simulink model "hwTarget"  (R2020b)
settings: Solver=VariableStepAuto  StartTime=0.0  StopTime=Ts  RelTol=1e-3
InitFcn:
  | evalin('base','pixelcontrolbus');
  | 
  | ROWS = 480;
  | COLS = 752;
  | 
  | OFFSET = 3;
  | imagesToRead = 20;
  | Ts = (imagesToRead + OFFSET) * 2;
  | 
  | inputNums = [1:imagesToRead];
  | 
  | MagThrL = 7;
  | MagThrS = 3;
  | SegMaxLength = 630;
  | 
  | NUM_OF_BITS = 32;
  | MSB = NUM_OF_BITS-1;
  | cap_1 = fixdt(0,NUM_OF_BITS,NUM_OF_BITS-1);
  | cap_2 = fixdt(0,NUM_OF_BITS,NUM_OF_BITS-2);
  | 
  | CORDIC_LUT_DT_1 = fixdt(1, NUM_OF_BITS, NUM_OF_BITS-2);
  | CORDIC_LUT_DT_2 = fixdt(1, NUM_OF_BITS, NUM_OF_BITS-1);
  | CORDIC_LUT_DT_3 = fixdt(1, NUM_OF_BITS, NUM_OF_BITS);
  | CORDIC_LUT_DT_4 = fixdt(1, NUM_OF_BITS, NUM_OF_BITS+1);
  | CORDIC_LUT_DT_5 = fixdt(1, NUM_OF_BITS, NUM_OF_BITS+1);
  | CORDIC_LUT_DT_6 = fixdt(1, NUM_OF_BITS, NUM_OF_BITS+2);
  | CORDIC_LUT_DT_7 = fixdt(1, NUM_OF_BITS, NUM_OF_BITS+3);
  | CORDIC_LUT_DT_8 = fixdt(1, NUM_OF_BITS, NUM_OF_BITS+4);
  | CORDIC_LUT_DT_9 = fixdt(1, NUM_OF_BITS, NUM_OF_BITS+5);
  | CORDIC_LUT_DT_10 = fixdt(1, NUM_OF_BITS, NUM_OF_BITS+6);
  | CORDIC_LUT_DT_11 = fixdt(1, NUM_OF_BITS, NUM_OF_BITS+7);
  | CORDIC_LUT_DT_12 = fixdt(1, NUM_OF_BITS, NUM_OF_BITS+8);
  | 
  | RGB_DT = fixdt(0, 24, 0);
  | GRAY_DT = fixdt(0, 8, 0);
  | THETA_DT = fixdt(1, 16, 13);
  | MAG_DT = fixdt(0, 16, 15);
  | KIRCH_DT = fixdt(0, 12, 0);
undefined symbols (not defined in the file or in its folder): bufferInit, bufferSize
libraries: hdlsllib x86, simulink x6, visionhdlstatistics x4, visionhdlio x2, visionhdlutilities x1
(part 1 of 3)
settings Model: Creator=tyson  LastModifiedBy=tyson

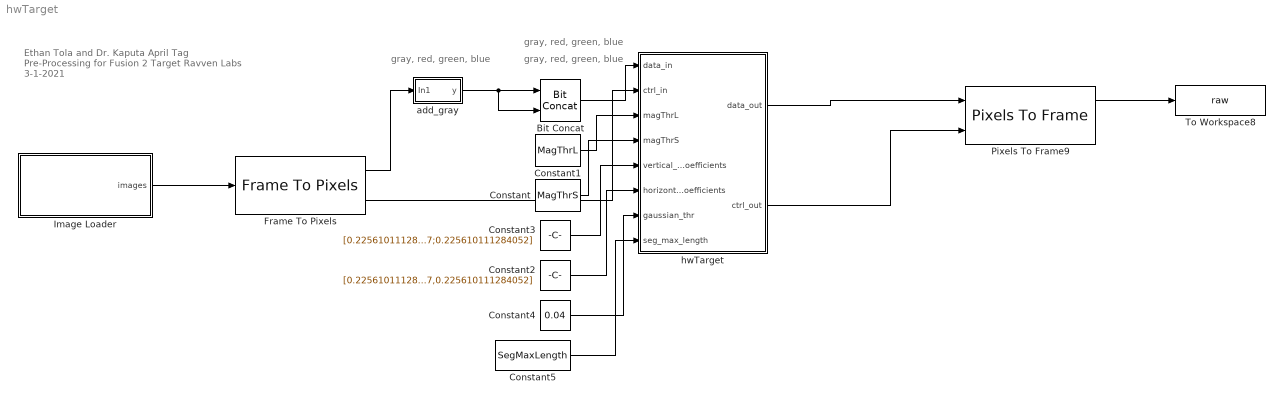
== system hwTarget ==
  note: Ethan Tola and Dr. Kaputa
      | April Tag Pre-Processing for Fusion 2 Target
      | Ravven Labs
      | 3-1-2021
  note: gray, red, green, blue
  note: gray, red, green, blue
  note: gray, red, green, blue
  Bit Concat : hdlsllib/Logic and Bit Operations/Bit Concat  numInputs=2
  Constant : Constant  Value=MagThrS  OutDataTypeStr=Inherit: Inherit via back propagation  SampleTime=-1
  Constant1 : Constant  Value=MagThrL  OutDataTypeStr=Inherit: Inherit via back propagation  SampleTime=-1
  Constant2 : Constant  Value=[0.225610111284052,0.548779777431897,0.225610111284052]  OutDataTypeStr=Inherit: Inherit via back propagation  SampleTime=-1
  Constant3 : Constant  Value=[0.225610111284051;0.548779777431897;0.225610111284052]  OutDataTypeStr=Inherit: Inherit via back propagation  SampleTime=-1
  Constant4 : Constant  Value=0.04  OutDataTypeStr=Inherit: Inherit via back propagation  SampleTime=-1
  Constant5 : Constant  Value=SegMaxLength
  Frame To Pixels : visionhdlio/Frame To Pixels  NumComponents=3  NumPixels=1  VideoFormat=Custom  ActivePixelsPerLine=752  ActiveVideoLines=480  TotalPixelsPerLine=752  TotalVideoLines=480  StartingActiveLine=1  FrontPorch=0  SampleTime=0
      settings: SourceProductName=Vision HDL Toolbox
  Image Loader : Subsystem
  Pixels To Frame9 : visionhdlio/Pixels To Frame  NumComponents=1  NumPixels=1  VideoFormat=Custom  ActivePixelsPerLine=752  ActiveVideoLines=480  TotalPixelsPerLine=752  TotalVideoLines=480
      settings: SourceProductBaseCode=VT
  To Workspace8 : ToWorkspace  VariableName=raw  SaveFormat=Timeseries  SampleTime=-1
  add_gray : Subsystem
  hwTarget : Subsystem  TreatAsAtomicUnit=on
  wires:
  Frame To Pixels/1 -> add_gray/1(In1)
  Bit Concat/1 -> hwTarget/1(data_in)
  hwTarget/1(data_out) -> Pixels To Frame9/1
  add_gray/1(y) -> Bit Concat/2, Bit Concat/1
  hwTarget/2(ctrl_out) -> Pixels To Frame9/2
  Frame To Pixels/2 -> hwTarget/2(ctrl_in)
  Pixels To Frame9/1 -> To Workspace8/1
  Image Loader/1(images) -> Frame To Pixels/1
  Constant1/1 -> hwTarget/3(magThrL)
  Constant/1 -> hwTarget/4(magThrS)
  Constant3/1 -> hwTarget/5(vertical_coefficients)
  Constant2/1 -> hwTarget/6(horizontal_coefficients)
  Constant4/1 -> hwTarget/7(gaussian_thr)
  Constant5/1 -> hwTarget/8(seg_max_length)

== system hwTarget/Image Loader ==
  Clock : Clock
  MATLAB Function : MATLAB Function  TreatAsAtomicUnit=on  SystemSampleTime=1
  images : Outport
  wires:
  Clock/1 -> MATLAB Function/1(simTime)
  MATLAB Function/1(images) -> images/1

== system hwTarget/add_gray ==
  note: Grayscale = (R * 0.25) + (G * 0.5) + (B * 0.125)
  In1 : Inport
  Bit Concat : hdlsllib/Logic and Bit Operations/Bit Concat  numInputs=4
  Demux : Demux  Outputs=3
  Shift Arithmetic3 : ArithShift  BitShiftNumber=1  BitShiftDirection=Right
  Shift Arithmetic4 : ArithShift  BitShiftNumber=2  BitShiftDirection=Right
  Shift Arithmetic5 : ArithShift  BitShiftNumber=3  BitShiftDirection=Right
  Sum : Sum  Inputs=+++  OutDataTypeStr=uint8
  y : Outport
  wires:
  Bit Concat/1 -> y/1
  In1/1 -> Demux/1
  Demux/2 -> Shift Arithmetic3/1, Bit Concat/3
  Demux/1 -> Shift Arithmetic4/1, Bit Concat/2
  Demux/3 -> Shift Arithmetic5/1, Bit Concat/4
  Sum/1 -> Bit Concat/1
  Shift Arithmetic4/1 -> Sum/1
  Shift Arithmetic3/1 -> Sum/2
  Shift Arithmetic5/1 -> Sum/3

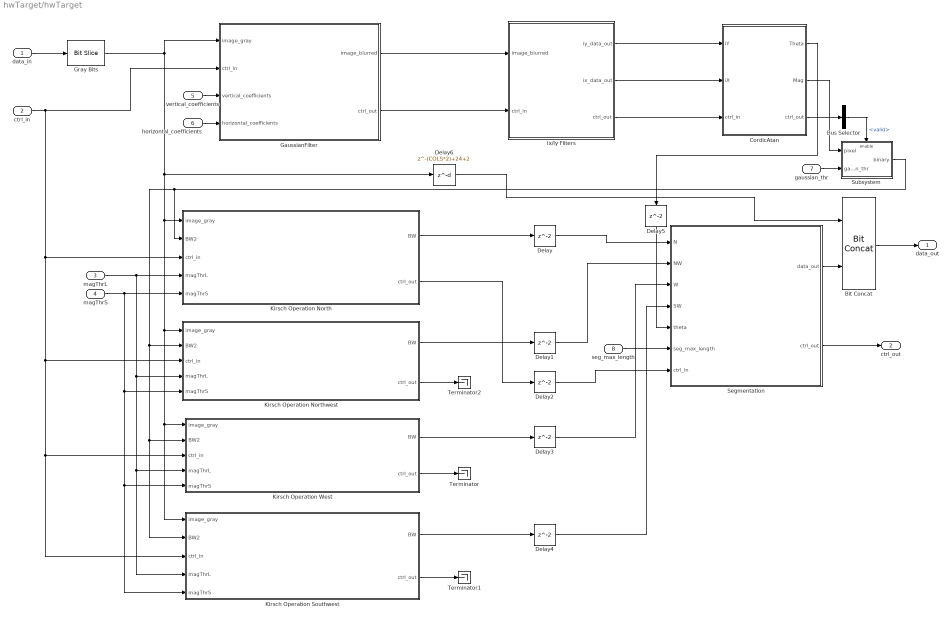
== system hwTarget/hwTarget ==
  data_in : Inport
  ctrl_in : Inport  Port=2
  magThrL : Inport  Port=3
  magThrS : Inport  Port=4
  vertical_coefficients : Inport  Port=5
  horizontal_coefficients : Inport  Port=6
  gaussian_thr : Inport  Port=7
  seg_max_length : Inport  Port=8
  Bit Concat : hdlsllib/Logic and Bit Operations/Bit Concat  numInputs=2
  Bus Selector : BusSelector  OutputSignals=valid
  CordicAtan : Subsystem
  Delay{,1..5} (6 alike) : Delay
  Delay6 : Delay  DelayLength=(COLS*2)+24+2
  GaussianFilter : Subsystem
  Gray Bits : hdlsllib/Logic and Bit Operations/Bit Slice  lidx=31  ridx=24
      settings: SourceProductBaseCode=SL
  Ix/Iy Filters : Subsystem
  Kirsch Operation North : Subsystem
  Kirsch Operation Northwest : Subsystem
  Kirsch Operation Southwest : Subsystem
  Kirsch Operation West : Subsystem
  Segmentation : Subsystem
  Subsystem : Subsystem
  Terminator : Terminator
  Terminator1 : Terminator
  Terminator2 : Terminator
  data_out : Outport
  ctrl_out : Outport  Port=2
  wires:
  Ix/Iy Filters/3(ctrl_out) -> CordicAtan/3(ctrl_in)
  GaussianFilter/2(ctrl_out) -> Ix/Iy Filters/2(ctrl_in)
  GaussianFilter/1(image_blurred) -> Ix/Iy Filters/1(image_blurred)
  Ix/Iy Filters/2(ix_data_out) -> CordicAtan/2(iX)
  Ix/Iy Filters/1(iy_data_out) -> CordicAtan/1(iY)
  data_in/1 -> Gray Bits/1
  CordicAtan/2(Mag) -> Subsystem/1(pixel)
  Bus Selector/1 -> Subsystem/Enable  "<valid>"
  ctrl_in/1 -> Kirsch Operation Southwest/3(ctrl_in), Kirsch Operation West/3(ctrl_in), Kirsch Operation Northwest/3(ctrl_in), Kirsch Operation North/3(ctrl_in), GaussianFilter/2(ctrl_in)
  Gray Bits/1 -> Delay6/1, Kirsch Operation Southwest/1(image_gray), Kirsch Operation West/1(image_gray), Kirsch Operation Northwest/1(image_gray), Kirsch Operation North/1(image_gray), GaussianFilter/1(image_gray)
  Subsystem/1(binary) -> Kirsch Operation North/2(BW2), Kirsch Operation Southwest/2(BW2), Kirsch Operation West/2(BW2), Kirsch Operation Northwest/2(BW2)
  CordicAtan/1(Theta) -> Delay5/1
  CordicAtan/3(ctrl_out) -> Bus Selector/1
  magThrL/1 -> Kirsch Operation Southwest/4(magThrL), Kirsch Operation West/4(magThrL), Kirsch Operation Northwest/4(magThrL), Kirsch Operation North/4(magThrL)
  magThrS/1 -> Kirsch Operation Southwest/5(magThrS), Kirsch Operation West/5(magThrS), Kirsch Operation Northwest/5(magThrS), Kirsch Operation North/5(magThrS)
  vertical_coefficients/1 -> GaussianFilter/3(vertical_coefficients)
  horizontal_coefficients/1 -> GaussianFilter/4(horizontal_coefficients)
  gaussian_thr/1 -> Subsystem/2(gaussian_thr)
  Kirsch Operation North/1(BW) -> Delay/1
  Kirsch Operation Northwest/1(BW) -> Delay1/1
  Kirsch Operation West/1(BW) -> Delay3/1
  Kirsch Operation Southwest/1(BW) -> Delay4/1
  Kirsch Operation North/2(ctrl_out) -> Delay2/1
  Delay/1 -> Segmentation/1(N)
  Delay1/1 -> Segmentation/2(NW)
  Delay2/1 -> Segmentation/7(ctrl_in)
  Delay3/1 -> Segmentation/3(W)
  Delay4/1 -> Segmentation/4(SW)
  Delay5/1 -> Segmentation/5(theta)
  Segmentation/2(ctrl_out) -> ctrl_out/1
  Kirsch Operation West/2(ctrl_out) -> Terminator/1
  Kirsch Operation Southwest/2(ctrl_out) -> Terminator1/1
  Kirsch Operation Northwest/2(ctrl_out) -> Terminator2/1
  Bit Concat/1 -> data_out/1
  Segmentation/1(data_out) -> Bit Concat/2
  Delay6/1 -> Bit Concat/1
  seg_max_length/1 -> Segmentation/6(seg_max_length)

== system hwTarget/hwTarget/CordicAtan ==
  iY : Inport
  iX : Inport  Port=2
  ctrl_in : Inport  Port=3
  Bus Selector : BusSelector  OutputSignals=valid
  CORDIC Algorithm : Subsystem
  Delay32 : Delay  DelayLength=14
  Theta : Outport
  Mag : Outport  Port=2
  ctrl_out : Outport  Port=3
  wires:
  Delay32/1 -> ctrl_out/1
  iY/1 -> CORDIC Algorithm/1(In1)
  iX/1 -> CORDIC Algorithm/2(In2)
  CORDIC Algorithm/1(Out1) -> Theta/1
  CORDIC Algorithm/2(Out2) -> Mag/1
  ctrl_in/1 -> Delay32/1, Bus Selector/1
  Bus Selector/1 -> CORDIC Algorithm/Enable  "<valid>"

== system hwTarget/hwTarget/GaussianFilter ==
  image_gray : Inport
  ctrl_in : Inport  Port=2
  vertical_coefficients : Inport  Port=3
  horizontal_coefficients : Inport  Port=4
  Bus Selector : BusSelector  OutputSignals=valid
  Data Type Duplicate : DataTypeDuplicate  NumInputPorts=3
  Delay1 : Delay  DelayLength=4
  Delay2 : Delay  DelayLength=4
  Normalize : Gain  Gain=1/255  OutDataTypeStr=cap_1
  Symmetric Filter : Subsystem
  image_blurred : Outport
  ctrl_out : Outport  Port=2
  wires:
  horizontal_coefficients/1 -> Data Type Duplicate/1, Symmetric Filter/2(horizontal_coefficients)
  ctrl_in/1 -> Delay1/1, Bus Selector/1
  Bus Selector/1 -> Symmetric Filter/Enable  "<valid>"
  vertical_coefficients/1 -> Data Type Duplicate/2, Symmetric Filter/1(verticle_coefficients)
  Delay1/1 -> Delay2/1
  Normalize/1 -> Data Type Duplicate/3, Symmetric Filter/3(data_in)
  image_gray/1 -> Normalize/1
  Delay2/1 -> ctrl_out/1
  Symmetric Filter/1(data_out) -> image_blurred/1

== system hwTarget/hwTarget/Ix//Iy Filters ==
  image_blurred : Inport
  ctrl_in : Inport  Port=2
  Delay1 : Delay
  Ix Filter : Subsystem
  Iy Filter : Subsystem
  iy_data_out : Outport
  ix_data_out : Outport  Port=2
  ctrl_out : Outport  Port=3
  wires:
  Iy Filter/1(data_out) -> iy_data_out/1
  image_blurred/1 -> Iy Filter/1(data_in), Ix Filter/1(data_in)
  Delay1/1 -> ctrl_out/1
  ctrl_in/1 -> Iy Filter/2(ctrl_in), Delay1/1, Ix Filter/2(ctrl_in)
  Ix Filter/1(data_out) -> ix_data_out/1

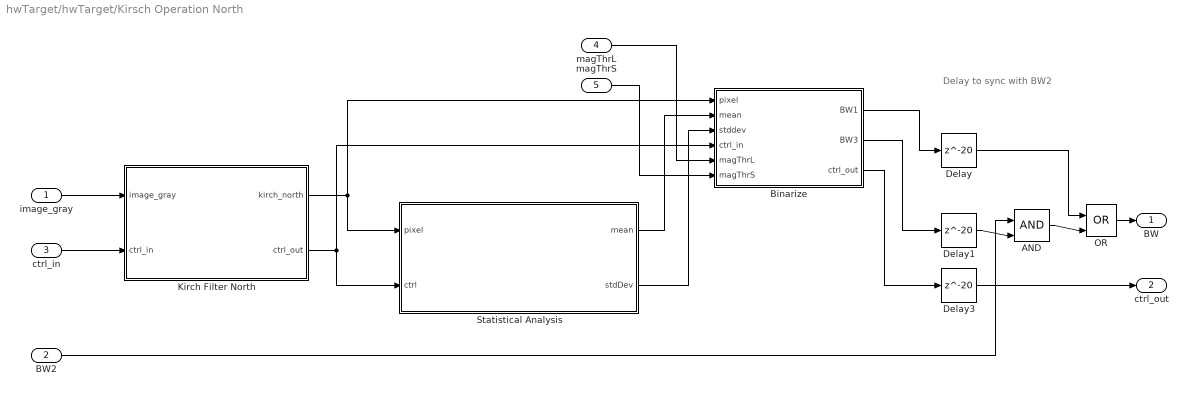
== system hwTarget/hwTarget/Kirsch Operation North ==
  note: Delay to sync with BW2
  image_gray : Inport
  BW2 : Inport  Port=2
  ctrl_in : Inport  Port=3
  magThrL : Inport  Port=4
  magThrS : Inport  Port=5
  AND : Logic  IconShape=distinctive  AllPortsSameDT=off  OutDataTypeStr=boolean
  Binarize : Subsystem
  Delay : Delay  DelayLength=20
  Delay1 : Delay  DelayLength=20
  Delay3 : Delay  DelayLength=20
  Kirch Filter North : Subsystem
  OR : Logic  Operator=OR  IconShape=distinctive  AllPortsSameDT=off  OutDataTypeStr=boolean
  Statistical Analysis : Subsystem
  BW : Outport
  ctrl_out : Outport  Port=2
  wires:
  Binarize/3(ctrl_out) -> Delay3/1
  Statistical Analysis/1(mean) -> Binarize/2(mean)
  Kirch Filter North/2(ctrl_out) -> Binarize/4(ctrl_in), Statistical Analysis/2(ctrl)
  Statistical Analysis/2(stdDev) -> Binarize/3(stddev)
  AND/1 -> OR/2
  Binarize/2(BW3) -> Delay1/1
  Delay/1 -> OR/1
  Binarize/1(BW1) -> Delay/1
  Delay1/1 -> AND/2
  OR/1 -> BW/1
  Delay3/1 -> ctrl_out/1
  BW2/1 -> AND/1
  ctrl_in/1 -> Kirch Filter North/2(ctrl_in)
  image_gray/1 -> Kirch Filter North/1(image_gray)
  Kirch Filter North/1(kirch_north) -> Binarize/1(pixel), Statistical Analysis/1(pixel)
  magThrS/1 -> Binarize/6(magThrS)
  magThrL/1 -> Binarize/5(magThrL)

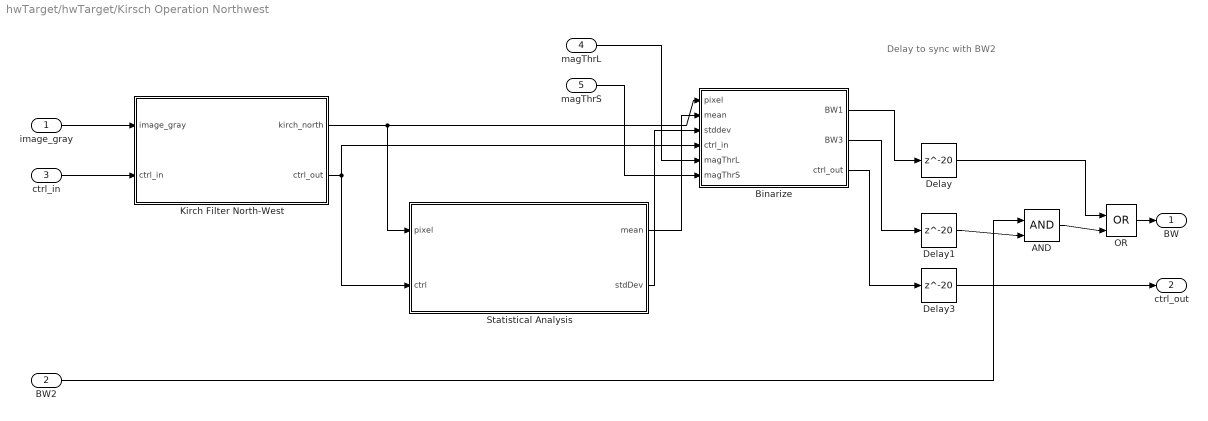
== system hwTarget/hwTarget/Kirsch Operation Northwest ==
  note: Delay to sync with BW2
  image_gray : Inport
  BW2 : Inport  Port=2
  ctrl_in : Inport  Port=3
  magThrL : Inport  Port=4
  magThrS : Inport  Port=5
  AND : Logic  IconShape=distinctive  AllPortsSameDT=off  OutDataTypeStr=boolean
  Binarize : Subsystem
  Delay : Delay  DelayLength=20
  Delay1 : Delay  DelayLength=20
  Delay3 : Delay  DelayLength=20
  Kirch Filter North-West : Subsystem
  OR : Logic  Operator=OR  IconShape=distinctive  AllPortsSameDT=off  OutDataTypeStr=boolean
  Statistical Analysis : Subsystem
  BW : Outport
  ctrl_out : Outport  Port=2
  wires:
  Delay1/1 -> AND/2
  Binarize/1(BW1) -> Delay/1
  Delay/1 -> OR/1
  Kirch Filter North-West/1(kirch_north) -> Binarize/1(pixel), Statistical Analysis/1(pixel)
  AND/1 -> OR/2
  Binarize/2(BW3) -> Delay1/1
  Binarize/3(ctrl_out) -> Delay3/1
  image_gray/1 -> Kirch Filter North-West/1(image_gray)
  Delay3/1 -> ctrl_out/1
  OR/1 -> BW/1
  Kirch Filter North-West/2(ctrl_out) -> Binarize/4(ctrl_in), Statistical Analysis/2(ctrl)
  ctrl_in/1 -> Kirch Filter North-West/2(ctrl_in)
  BW2/1 -> AND/1
  magThrS/1 -> Binarize/6(magThrS)
  magThrL/1 -> Binarize/5(magThrL)
  Statistical Analysis/2(stdDev) -> Binarize/3(stddev)
  Statistical Analysis/1(mean) -> Binarize/2(mean)

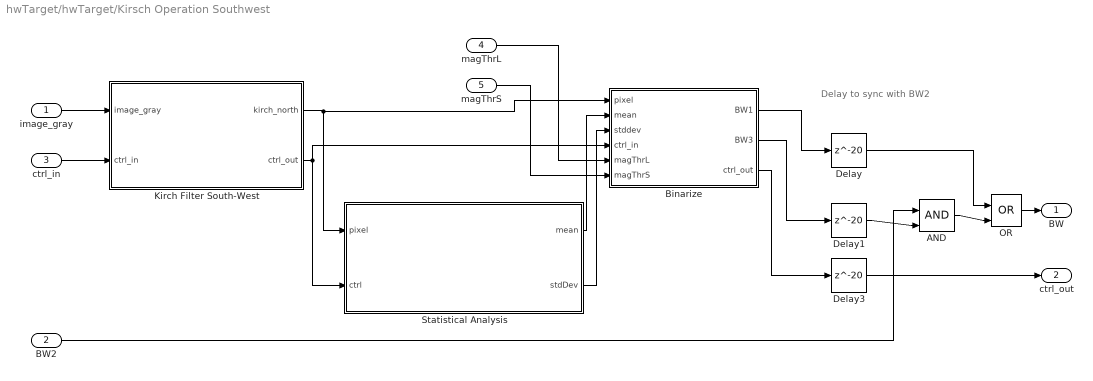
== system hwTarget/hwTarget/Kirsch Operation Southwest ==
  note: Delay to sync with BW2
  image_gray : Inport
  BW2 : Inport  Port=2
  ctrl_in : Inport  Port=3
  magThrL : Inport  Port=4
  magThrS : Inport  Port=5
  AND : Logic  IconShape=distinctive  AllPortsSameDT=off  OutDataTypeStr=boolean
  Binarize : Subsystem
  Delay : Delay  DelayLength=20
  Delay1 : Delay  DelayLength=20
  Delay3 : Delay  DelayLength=20
  Kirch Filter South-West : Subsystem
  OR : Logic  Operator=OR  IconShape=distinctive  AllPortsSameDT=off  OutDataTypeStr=boolean
  Statistical Analysis : Subsystem
  BW : Outport
  ctrl_out : Outport  Port=2
  wires:
  Delay/1 -> OR/1
  Kirch Filter South-West/1(kirch_north) -> Binarize/1(pixel), Statistical Analysis/1(pixel)
  Statistical Analysis/1(mean) -> Binarize/2(mean)
  Binarize/3(ctrl_out) -> Delay3/1
  OR/1 -> BW/1
  Kirch Filter South-West/2(ctrl_out) -> Binarize/4(ctrl_in), Statistical Analysis/2(ctrl)
  AND/1 -> OR/2
  Binarize/2(BW3) -> Delay1/1
  Statistical Analysis/2(stdDev) -> Binarize/3(stddev)
  Binarize/1(BW1) -> Delay/1
  Delay1/1 -> AND/2
  ctrl_in/1 -> Kirch Filter South-West/2(ctrl_in)
  image_gray/1 -> Kirch Filter South-West/1(image_gray)
  BW2/1 -> AND/1
  Delay3/1 -> ctrl_out/1
  magThrL/1 -> Binarize/5(magThrL)
  magThrS/1 -> Binarize/6(magThrS)

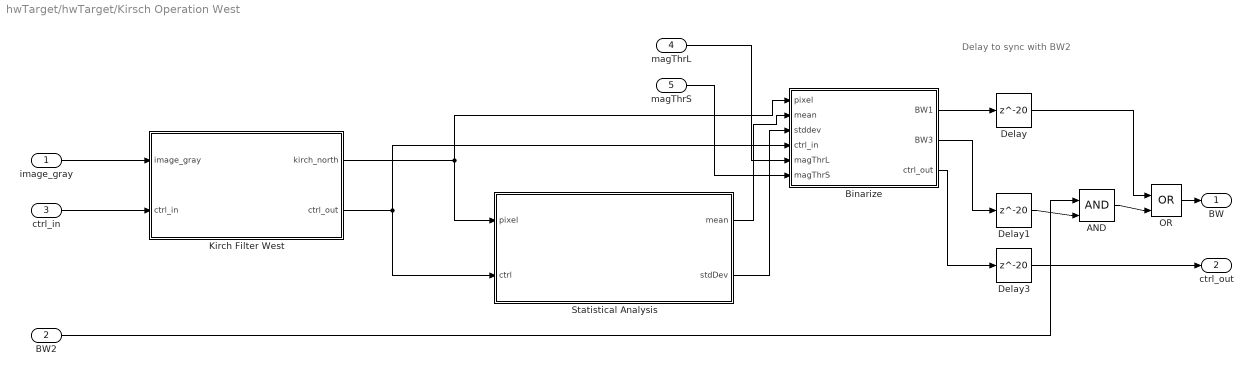
== system hwTarget/hwTarget/Kirsch Operation West ==
  note: Delay to sync with BW2
  image_gray : Inport
  BW2 : Inport  Port=2
  ctrl_in : Inport  Port=3
  magThrL : Inport  Port=4
  magThrS : Inport  Port=5
  AND : Logic  IconShape=distinctive  AllPortsSameDT=off  OutDataTypeStr=boolean
  Binarize : Subsystem
  Delay : Delay  DelayLength=20
  Delay1 : Delay  DelayLength=20
  Delay3 : Delay  DelayLength=20
  Kirch Filter West : Subsystem
  OR : Logic  Operator=OR  IconShape=distinctive  AllPortsSameDT=off  OutDataTypeStr=boolean
  Statistical Analysis : Subsystem
  BW : Outport
  ctrl_out : Outport  Port=2
  wires:
  Statistical Analysis/2(stdDev) -> Binarize/3(stddev)
  Binarize/3(ctrl_out) -> Delay3/1
  Statistical Analysis/1(mean) -> Binarize/2(mean)
  Binarize/2(BW3) -> Delay1/1
  Delay/1 -> OR/1
  Kirch Filter West/2(ctrl_out) -> Binarize/4(ctrl_in), Statistical Analysis/2(ctrl)
  AND/1 -> OR/2
  Binarize/1(BW1) -> Delay/1
  Kirch Filter West/1(kirch_north) -> Binarize/1(pixel), Statistical Analysis/1(pixel)
  Delay1/1 -> AND/2
  image_gray/1 -> Kirch Filter West/1(image_gray)
  Delay3/1 -> ctrl_out/1
  ctrl_in/1 -> Kirch Filter West/2(ctrl_in)
  OR/1 -> BW/1
  BW2/1 -> AND/1
  magThrL/1 -> Binarize/5(magThrL)
  magThrS/1 -> Binarize/6(magThrS)

== system hwTarget/hwTarget/Segmentation ==
  N : Inport
  NW : Inport  Port=2
  W : Inport  Port=3
  SW : Inport  Port=4
  theta : Inport  Port=5
  seg_max_length : Inport  Port=6
  ctrl_in : Inport  Port=7
  North Segmentation : Subsystem  TreatAsAtomicUnit=on
  Northwest Segmentation : Subsystem
  Southwest Segmentation : Subsystem
  West Segmentation : Subsystem
  data_out : Outport
  ctrl_out : Outport  Port=2
  wires:
  N/1 -> North Segmentation/1(pixel_in)
  theta/1 -> North Segmentation/2(theta)
  ctrl_in/1 -> North Segmentation/3(ctrl_in)
  North Segmentation/1(pixel_out) -> data_out/1
  North Segmentation/2(ctrl_out) -> ctrl_out/1

== system hwTarget/hwTarget/Subsystem ==
  pixel : Inport
  gaussian_thr : Inport  Port=2
  Enable : EnablePort
  Comparator1 : RelationalOperator  Operator=>  OutDataTypeStr=boolean  RndMeth=Simplest
  Data Type Duplicate : DataTypeDuplicate
  binary : Outport
  wires:
  Comparator1/1 -> binary/1
  gaussian_thr/1 -> Data Type Duplicate/2, Comparator1/2
  pixel/1 -> Data Type Duplicate/1, Comparator1/1

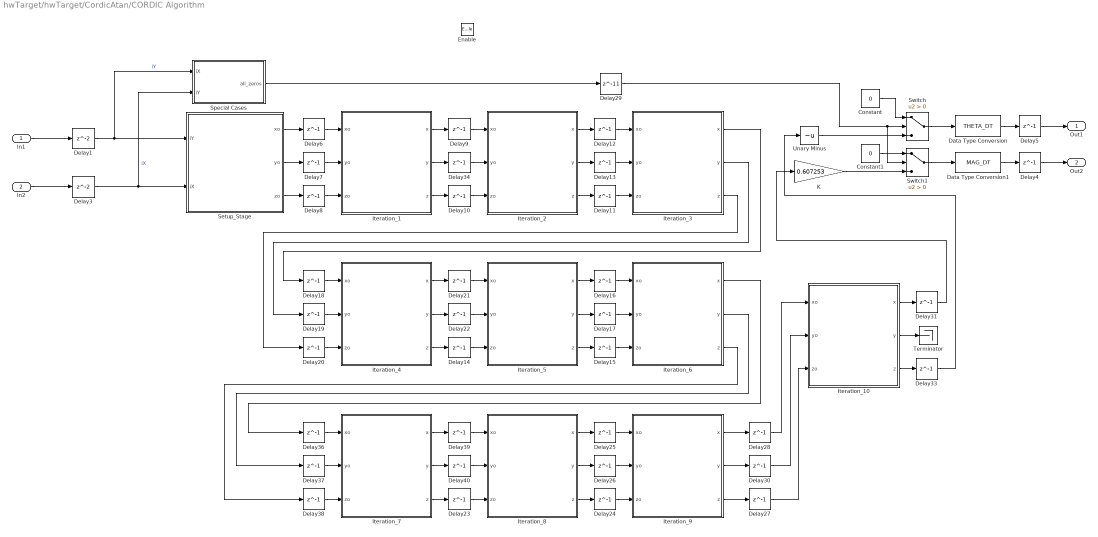
== system hwTarget/hwTarget/CordicAtan/CORDIC Algorithm ==
  In1 : Inport
  In2 : Inport  Port=2
  Enable : EnablePort
  Constant : Constant  Value=0  OutDataTypeStr=Inherit: Inherit via back propagation  SampleTime=-1
  Constant1 : Constant  Value=0  OutDataTypeStr=Inherit: Inherit via back propagation  SampleTime=-1
  Data Type Conversion : DataTypeConversion  OutDataTypeStr=THETA_DT
  Data Type Conversion1 : DataTypeConversion  OutDataTypeStr=MAG_DT
  Delay1 : Delay
  Delay{4..28,30..31,33..34,36..40} (34 alike) : Delay  DelayLength=1
  Delay29 : Delay  DelayLength=11
  Delay3 : Delay
  Iteration_1 : Subsystem
  Iteration_10 : Subsystem
  Iteration_2 : Subsystem
  Iteration_3 : Subsystem
  Iteration_4 : Subsystem
  Iteration_5 : Subsystem
  Iteration_6 : Subsystem
  Iteration_7 : Subsystem
  Iteration_8 : Subsystem
  Iteration_9 : Subsystem
  K : Gain  Gain=0.607253  OutDataTypeStr=fixdt(0,32, 31)
  Setup_Stage : Subsystem
  Special Cases : Subsystem
  Switch : Switch  Criteria=u2 > Threshold
  Switch1 : Switch  Criteria=u2 > Threshold
  Terminator : Terminator
  Unary Minus : UnaryMinus
  Out1 : Outport
  Out2 : Outport  Port=2
  wires:
  Delay12/1 -> Iteration_3/1(xo)
  Iteration_9/1(x) -> Delay28/1
  Delay30/1 -> Iteration_10/2(yo)
  Iteration_6/3(z) -> Delay38/1
  Iteration_1/1(x) -> Delay9/1
  Iteration_3/3(z) -> Delay20/1
  Delay3/1 -> Special Cases/2(iY), Setup_Stage/2(iX)  "iX"
  Iteration_8/2(y) -> Delay26/1
  K/1 -> Switch1/3
  Delay11/1 -> Iteration_3/3(zo)
  Delay13/1 -> Iteration_3/2(yo)
  Delay21/1 -> Iteration_5/1(xo)
  Setup_Stage/2(yo) -> Delay7/1
  Iteration_10/3(z) -> Delay33/1
  Delay29/1 -> Switch1/2, Switch/2
  Delay31/1 -> K/1
  Delay33/1 -> Unary Minus/1
  Delay16/1 -> Iteration_6/1(xo)
  Delay17/1 -> Iteration_6/2(yo)
  Delay9/1 -> Iteration_2/1(xo)
  Iteration_2/3(z) -> Delay11/1
  Delay28/1 -> Iteration_10/1(xo)
  Delay20/1 -> Iteration_4/3(zo)
  Delay22/1 -> Iteration_5/2(yo)
  Delay8/1 -> Iteration_1/3(zo)
  Iteration_3/1(x) -> Delay18/1
  Data Type Conversion1/1 -> Delay4/1
  Iteration_4/3(z) -> Delay14/1
  Delay23/1 -> Iteration_8/3(zo)
  Delay18/1 -> Iteration_4/1(xo)
  Delay40/1 -> Iteration_8/2(yo)
  Iteration_5/2(y) -> Delay17/1
  Iteration_7/2(y) -> Delay40/1
  Setup_Stage/3(zo) -> Delay8/1
  Delay34/1 -> Iteration_2/2(yo)
  Iteration_9/2(y) -> Delay30/1
  Delay25/1 -> Iteration_9/1(xo)
  Iteration_5/1(x) -> Delay16/1
  Iteration_1/3(z) -> Delay10/1
  Delay7/1 -> Iteration_1/2(yo)
  Iteration_7/3(z) -> Delay23/1
  Delay15/1 -> Iteration_6/3(zo)
  Iteration_2/1(x) -> Delay12/1
  Special Cases/1(all_zeros) -> Delay29/1
  Setup_Stage/1(xo) -> Delay6/1
  Delay6/1 -> Iteration_1/1(xo)
  Iteration_4/1(x) -> Delay21/1
  Data Type Conversion/1 -> Delay5/1
  Iteration_3/2(y) -> Delay19/1
  Iteration_4/2(y) -> Delay22/1
  Iteration_6/2(y) -> Delay37/1
  Iteration_9/3(z) -> Delay27/1
  Delay39/1 -> Iteration_8/1(xo)
  Iteration_2/2(y) -> Delay13/1
  Iteration_8/1(x) -> Delay25/1
  Iteration_1/2(y) -> Delay34/1
  Delay10/1 -> Iteration_2/3(zo)
  Iteration_8/3(z) -> Delay24/1
  Delay38/1 -> Iteration_7/3(zo)
  Delay26/1 -> Iteration_9/2(yo)
  Iteration_7/1(x) -> Delay39/1
  Delay19/1 -> Iteration_4/2(yo)
  Iteration_10/2(y) -> Terminator/1
  Iteration_6/1(x) -> Delay36/1
  Delay1/1 -> Special Cases/1(iX), Setup_Stage/1(iY)  "iY"
  Delay36/1 -> Iteration_7/1(xo)
  Iteration_5/3(z) -> Delay15/1
  Delay37/1 -> Iteration_7/2(yo)
  Delay24/1 -> Iteration_9/3(zo)
  Unary Minus/1 -> Switch/3
  Delay27/1 -> Iteration_10/3(zo)
  Constant/1 -> Switch/1
  Delay14/1 -> Iteration_5/3(zo)
  Iteration_10/1(x) -> Delay31/1
  Switch1/1 -> Data Type Conversion1/1
  Switch/1 -> Data Type Conversion/1
  Constant1/1 -> Switch1/1
  In1/1 -> Delay1/1
  In2/1 -> Delay3/1
  Delay5/1 -> Out1/1
  Delay4/1 -> Out2/1

== system hwTarget/hwTarget/GaussianFilter/Symmetric Filter ==
  verticle_coefficients : Inport
  horizontal_coefficients : Inport  Port=2
  data_in : Inport  Port=3
  Enable : EnablePort
  Mux : Mux  Inputs=3
  Row Filter1 : Subsystem
  Row Filter2 : Subsystem
  Row Filter3 : Subsystem
  Verticle Filter : Subsystem
  slicer : Subsystem
  data_out : Outport  InitialOutput=0
  wires:
  Row Filter2/1(data_out) -> Mux/2
  Row Filter3/1(data_out) -> Mux/3
  Row Filter1/1(data_out) -> Mux/1
  slicer/1(Row1) -> Row Filter1/1(data_in)
  data_in/1 -> slicer/1(data_in)
  horizontal_coefficients/1 -> Row Filter3/2(coefficients), Row Filter2/2(coefficients), Row Filter1/2(coefficients)
  slicer/2(Row2) -> Row Filter2/1(data_in)
  slicer/3(Row3) -> Row Filter3/1(data_in)
  Mux/1 -> Verticle Filter/1(data_in)
  Verticle Filter/1(data_out) -> data_out/1
  verticle_coefficients/1 -> Verticle Filter/2(coefficients)

== system hwTarget/hwTarget/Ix//Iy Filters/Ix Filter ==
  data_in : Inport
  ctrl_in : Inport  Port=2
  Bus Selector : BusSelector  OutputSignals=valid
  Filter : Subsystem
  data_out : Outport
  wires:
  ctrl_in/1 -> Bus Selector/1
  data_in/1 -> Filter/1(data_in)
  Filter/1(data_out) -> data_out/1
  Bus Selector/1 -> Filter/Enable  "<valid>"

== system hwTarget/hwTarget/Ix//Iy Filters/Iy Filter ==
  data_in : Inport
  ctrl_in : Inport  Port=2
  Bus Selector : BusSelector  OutputSignals=valid
  Filter : Subsystem
  data_out : Outport
  wires:
  ctrl_in/1 -> Bus Selector/1
  data_in/1 -> Filter/1(data_in)
  Filter/1(data_out) -> data_out/1
  Bus Selector/1 -> Filter/Enable  "<valid>"

== system hwTarget/hwTarget/Kirsch Operation North/Binarize ==
  pixel : Inport
  mean : Inport  Port=2
  stddev : Inport  Port=3
  ctrl_in : Inport  Port=4
  magThrL : Inport  Port=5
  magThrS : Inport  Port=6
  Bus Selector : BusSelector  OutputSignals=valid
  Delay : Delay  DelayLength=1
  Subsystem : Subsystem
  BW1 : Outport
  BW3 : Outport  Port=2
  ctrl_out : Outport  Port=3
  wires:
  pixel/1 -> Subsystem/1(pixel)
  mean/1 -> Subsystem/2(mean)
  stddev/1 -> Subsystem/3(stddev)
  Subsystem/1(Out1) -> BW1/1
  Subsystem/2(Out2) -> BW3/1
  ctrl_in/1 -> Delay/1, Bus Selector/1
  Bus Selector/1 -> Subsystem/Enable  "<valid>"
  Delay/1 -> ctrl_out/1
  magThrL/1 -> Subsystem/4(magThrL)
  magThrS/1 -> Subsystem/5(magThrS)

== system hwTarget/hwTarget/Kirsch Operation North/Kirch Filter North ==
  image_gray : Inport
  ctrl_in : Inport  Port=2
  Bus Selector : BusSelector  OutputSignals=valid
  Delay4 : Delay  DelayLength=3
  Kirch Filter : Subsystem
  kirch_north : Outport
  ctrl_out : Outport  Port=2
  wires:
  Delay4/1 -> ctrl_out/1
  ctrl_in/1 -> Bus Selector/1, Delay4/1
  image_gray/1 -> Kirch Filter/1(data_in)
  Kirch Filter/1(Out1) -> kirch_north/1
  Bus Selector/1 -> Kirch Filter/Enable  "<valid>"

== system hwTarget/hwTarget/Kirsch Operation North/Statistical Analysis ==
  pixel : Inport
  ctrl : Inport  Port=2
  Constant4 : Constant  SampleTime=-1
  Image Statistics : visionhdlstatistics/Image Statistics  mean=on  variance=off  stdDev=on  SimulateUsing=Code generation
      settings: SourceProductBaseCode=VT
  Latch : Subsystem
  Latch1 : Subsystem
  mean : Outport
  stdDev : Outport  Port=2
  wires:
  Constant4/1 -> Latch1/3(rstn), Latch/3(rstn)
  Latch1/1(Q) -> stdDev/1
  Image Statistics/1 -> Latch/1(D)
  Image Statistics/3 -> Latch/2(en), Latch1/2(en)
  ctrl/1 -> Image Statistics/2
  Image Statistics/2 -> Latch1/1(D)
  pixel/1 -> Image Statistics/1
  Latch/1(Q) -> mean/1

== system hwTarget/hwTarget/Kirsch Operation Northwest/Binarize ==
  pixel : Inport
  mean : Inport  Port=2
  stddev : Inport  Port=3
  ctrl_in : Inport  Port=4
  magThrL : Inport  Port=5
  magThrS : Inport  Port=6
  Bus Selector : BusSelector  OutputSignals=valid
  Delay : Delay  DelayLength=1
  Subsystem : Subsystem
  BW1 : Outport
  BW3 : Outport  Port=2
  ctrl_out : Outport  Port=3
  wires:
  pixel/1 -> Subsystem/1(pixel)
  mean/1 -> Subsystem/2(mean)
  stddev/1 -> Subsystem/3(stddev)
  Subsystem/1(Out1) -> BW1/1
  Subsystem/2(Out2) -> BW3/1
  ctrl_in/1 -> Delay/1, Bus Selector/1
  Bus Selector/1 -> Subsystem/Enable  "<valid>"
  Delay/1 -> ctrl_out/1
  magThrL/1 -> Subsystem/4(magThrL)
  magThrS/1 -> Subsystem/5(magThrS)

== system hwTarget/hwTarget/Kirsch Operation Northwest/Kirch Filter North-West ==
  image_gray : Inport
  ctrl_in : Inport  Port=2
  Bus Selector : BusSelector  OutputSignals=valid
  Delay4 : Delay  DelayLength=3
  Kirch Filter : Subsystem
  kirch_north : Outport
  ctrl_out : Outport  Port=2
  wires:
  Delay4/1 -> ctrl_out/1
  ctrl_in/1 -> Delay4/1, Bus Selector/1
  image_gray/1 -> Kirch Filter/1(data_in)
  Kirch Filter/1(Out1) -> kirch_north/1
  Bus Selector/1 -> Kirch Filter/Enable  "<valid>"

== system hwTarget/hwTarget/Kirsch Operation Northwest/Statistical Analysis ==
  pixel : Inport
  ctrl : Inport  Port=2
  Constant4 : Constant  SampleTime=-1
  Image Statistics : visionhdlstatistics/Image Statistics  mean=on  variance=off  stdDev=on  SimulateUsing=Code generation
      settings: SourceProductBaseCode=VT
  Latch : Subsystem
  Latch1 : Subsystem
  mean : Outport
  stdDev : Outport  Port=2
  wires:
  Constant4/1 -> Latch1/3(rstn), Latch/3(rstn)
  Latch1/1(Q) -> stdDev/1
  Image Statistics/1 -> Latch/1(D)
  Image Statistics/3 -> Latch/2(en), Latch1/2(en)
  ctrl/1 -> Image Statistics/2
  Image Statistics/2 -> Latch1/1(D)
  pixel/1 -> Image Statistics/1
  Latch/1(Q) -> mean/1

== system hwTarget/hwTarget/Kirsch Operation Southwest/Binarize ==
  pixel : Inport
  mean : Inport  Port=2
  stddev : Inport  Port=3
  ctrl_in : Inport  Port=4
  magThrL : Inport  Port=5
  magThrS : Inport  Port=6
  Bus Selector : BusSelector  OutputSignals=valid
  Delay : Delay  DelayLength=1
  Subsystem : Subsystem
  BW1 : Outport
  BW3 : Outport  Port=2
  ctrl_out : Outport  Port=3
  wires:
  pixel/1 -> Subsystem/1(pixel)
  mean/1 -> Subsystem/2(mean)
  stddev/1 -> Subsystem/3(stddev)
  Subsystem/1(Out1) -> BW1/1
  Subsystem/2(Out2) -> BW3/1
  ctrl_in/1 -> Delay/1, Bus Selector/1
  Bus Selector/1 -> Subsystem/Enable  "<valid>"
  Delay/1 -> ctrl_out/1
  magThrL/1 -> Subsystem/4(magThrL)
  magThrS/1 -> Subsystem/5(magThrS)

== system hwTarget/hwTarget/Kirsch Operation Southwest/Kirch Filter South-West ==
  image_gray : Inport
  ctrl_in : Inport  Port=2
  Bus Selector : BusSelector  OutputSignals=valid
  Delay4 : Delay  DelayLength=3
  Subsystem : Subsystem
  kirch_north : Outport
  ctrl_out : Outport  Port=2
  wires:
  Delay4/1 -> ctrl_out/1
  ctrl_in/1 -> Bus Selector/1, Delay4/1
  image_gray/1 -> Subsystem/1(data_in)
  Subsystem/1(Out1) -> kirch_north/1
  Bus Selector/1 -> Subsystem/Enable  "<valid>"

== system hwTarget/hwTarget/Kirsch Operation Southwest/Statistical Analysis ==
  pixel : Inport
  ctrl : Inport  Port=2
  Constant4 : Constant  SampleTime=-1
  Image Statistics : visionhdlstatistics/Image Statistics  mean=on  variance=off  stdDev=on  SimulateUsing=Code generation
      settings: SourceProductBaseCode=VT
  Latch : Subsystem
  Latch1 : Subsystem
  mean : Outport
  stdDev : Outport  Port=2
  wires:
  Constant4/1 -> Latch1/3(rstn), Latch/3(rstn)
  Latch1/1(Q) -> stdDev/1
  Image Statistics/1 -> Latch/1(D)
  Image Statistics/3 -> Latch/2(en), Latch1/2(en)
  ctrl/1 -> Image Statistics/2
  Image Statistics/2 -> Latch1/1(D)
  pixel/1 -> Image Statistics/1
  Latch/1(Q) -> mean/1

== system hwTarget/hwTarget/Kirsch Operation West/Binarize ==
  pixel : Inport
  mean : Inport  Port=2
  stddev : Inport  Port=3
  ctrl_in : Inport  Port=4
  magThrL : Inport  Port=5
  magThrS : Inport  Port=6
  Bus Selector : BusSelector  OutputSignals=valid
  Delay : Delay  DelayLength=1
  Subsystem : Subsystem
  BW1 : Outport
  BW3 : Outport  Port=2
  ctrl_out : Outport  Port=3
  wires:
  pixel/1 -> Subsystem/1(pixel)
  mean/1 -> Subsystem/2(mean)
  stddev/1 -> Subsystem/3(stddev)
  Subsystem/1(Out1) -> BW1/1
  Subsystem/2(Out2) -> BW3/1
  ctrl_in/1 -> Delay/1, Bus Selector/1
  Bus Selector/1 -> Subsystem/Enable  "<valid>"
  Delay/1 -> ctrl_out/1
  magThrL/1 -> Subsystem/4(magThrL)
  magThrS/1 -> Subsystem/5(magThrS)

== system hwTarget/hwTarget/Kirsch Operation West/Kirch Filter West ==
  image_gray : Inport
  ctrl_in : Inport  Port=2
  Bus Selector : BusSelector  OutputSignals=valid
  Delay4 : Delay  DelayLength=3
  Subsystem : Subsystem
  kirch_north : Outport
  ctrl_out : Outport  Port=2
  wires:
  Delay4/1 -> ctrl_out/1
  ctrl_in/1 -> Bus Selector/1, Delay4/1
  image_gray/1 -> Subsystem/1(data_in)
  Subsystem/1(Out1) -> kirch_north/1
  Bus Selector/1 -> Subsystem/Enable  "<valid>"

== system hwTarget/hwTarget/Kirsch Operation West/Statistical Analysis ==
  pixel : Inport
  ctrl : Inport  Port=2
  Constant4 : Constant  SampleTime=-1
  Image Statistics : visionhdlstatistics/Image Statistics  mean=on  variance=off  stdDev=on  SimulateUsing=Code generation
      settings: SourceProductBaseCode=VT
  Latch : Subsystem
  Latch1 : Subsystem
  mean : Outport
  stdDev : Outport  Port=2
  wires:
  Constant4/1 -> Latch1/3(rstn), Latch/3(rstn)
  Latch1/1(Q) -> stdDev/1
  Image Statistics/1 -> Latch/1(D)
  Image Statistics/3 -> Latch/2(en), Latch1/2(en)
  ctrl/1 -> Image Statistics/2
  Image Statistics/2 -> Latch1/1(D)
  pixel/1 -> Image Statistics/1
  Latch/1(Q) -> mean/1

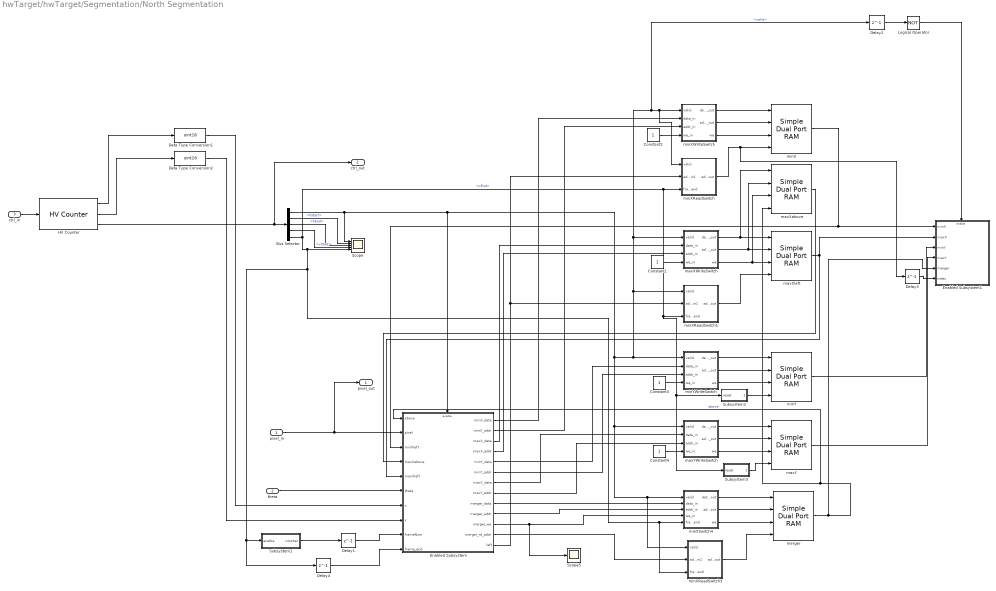
== system hwTarget/hwTarget/Segmentation/North Segmentation ==
  pixel_in : Inport
  theta : Inport  Port=2
  ctrl_in : Inport  Port=3
  Bus Selector : BusSelector  OutputSignals=valid,hStart,hEnd,vStart,vEnd
  Constant{1..4} (4 alike) : Constant  OutDataTypeStr=boolean  SampleTime=-1
  Data Type Conversion1 : DataTypeConversion  OutDataTypeStr=uint16
  Data Type Conversion2 : DataTypeConversion  OutDataTypeStr=uint16
  Delay{1..4} (4 alike) : Delay  DelayLength=1  InitialCondition=0
  Enabled Subsystem : Subsystem  TreatAsAtomicUnit=on
  Enabled Subsystem1 : Subsystem  TreatAsAtomicUnit=on
  HV Counter : visionhdlutilities/HV Counter  ActivePixelsPerLine=320  ActiveVideoLines=240  SimulateUsing=Code generation
      settings: SourceProductBaseCode=VT
  Logical Operator : Logic  Operator=NOT  AllPortsSameDT=off  OutDataTypeStr=boolean
  Scope : Scope  NumInputPorts=5
  Scope5 : Scope
  Subsystem1 : Subsystem
  Subsystem2 : Subsystem
  Subsystem3 : Subsystem
  maxXWriteSwitch : Subsystem
  maxXabove : hdlsllib/HDL RAMs/Simple Dual Port RAM  ram_size=16
      settings: SourceProductBaseCode=SL
  maxXleft : hdlsllib/HDL RAMs/Simple Dual Port RAM  ram_size=16
      settings: SourceProductBaseCode=SL
  maxY : hdlsllib/HDL RAMs/Simple Dual Port RAM  ram_size=16
      settings: SourceProductBaseCode=SL
  maxYWriteSwitch : Subsystem
  merger : hdlsllib/HDL RAMs/Simple Dual Port RAM  ram_size=16
      settings: SourceProductBaseCode=SL
  minX : hdlsllib/HDL RAMs/Simple Dual Port RAM  ram_size=16
      settings: SourceProductBaseCode=SL
  minXReadSwitch : Subsystem
  minXReadSwitch1 : Subsystem
  minXReadSwitch3 : Subsystem
  minXSwitch4 : Subsystem
  minXWriteSwitch : Subsystem
  minY : hdlsllib/HDL RAMs/Simple Dual Port RAM  ram_size=16
      settings: SourceProductBaseCode=SL
  minYWriteSwitch : Subsystem
  pixel_out : Outport
  ctrl_out : Outport  Port=2
  wires:
  Bus Selector/1 -> Scope/1, Enabled Subsystem/Enable, minYWriteSwitch/1(valid), minXReadSwitch1/1(valid), maxXWriteSwitch/1(valid), Delay2/1, minXReadSwitch/1(valid), minXWriteSwitch/1(valid), minXReadSwitch3/1(valid), minXSwitch4/1(valid), maxYWriteSwitch/1(valid)  "<valid>"
  minXWriteSwitch/2(addr_out) -> minX/2
  minYWriteSwitch/1(data_out) -> minY/1
  maxXWriteSwitch/3(we) -> maxXabove/3, maxXleft/3
  minXSwitch4/2(addr_out) -> merger/2
  minXSwitch4/3(we) -> merger/3
  minXSwitch4/1(data_out) -> merger/1
  minXWriteSwitch/1(data_out) -> minX/1
  minYWriteSwitch/2(addr_out) -> minY/2
  maxYWriteSwitch/1(data_out) -> maxY/1
  minXWriteSwitch/3(we) -> minX/3
  maxYWriteSwitch/2(addr_out) -> maxY/2
  merger/1 -> Enabled Subsystem1/5(merger), Enabled Subsystem/1(above), maxXabove/4  "above"
  maxXWriteSwitch/1(data_out) -> maxXabove/1, maxXleft/1
  maxYWriteSwitch/3(we) -> maxY/3
  maxXWriteSwitch/2(addr_out) -> maxXabove/2, maxXleft/2
  minYWriteSwitch/3(we) -> minY/3
  ctrl_in/1 -> HV Counter/1
  HV Counter/2 -> Data Type Conversion2/1
  HV Counter/1 -> Data Type Conversion1/1
  Data Type Conversion1/1 -> Enabled Subsystem/7(x)
  Enabled Subsystem/9(merger_data) -> minXSwitch4/2(data_in)
  Enabled Subsystem/10(merger_addr) -> minXSwitch4/3(addr_in)
  Enabled Subsystem/11(merger_we) -> Scope5/1, minXSwitch4/4(we_in)
  Enabled Subsystem/7(maxY_data) -> maxYWriteSwitch/2(data_in)
  Enabled Subsystem/8(maxY_addr) -> maxYWriteSwitch/3(addr_in)
  Enabled Subsystem/6(minY_addr) -> minYWriteSwitch/3(addr_in)
  Enabled Subsystem/5(minY_data) -> minYWriteSwitch/2(data_in)
  Enabled Subsystem/4(maxX_addr) -> maxXWriteSwitch/3(addr_in)
  Enabled Subsystem/3(maxX_data) -> maxXWriteSwitch/2(data_in)
  Enabled Subsystem/2(minX_addr) -> minXWriteSwitch/3(addr_in)
  Enabled Subsystem/1(minX_data) -> minXWriteSwitch/2(data_in)
  maxXabove/1 -> Enabled Subsystem/4(maxXabove)
  maxXleft/1 -> Enabled Subsystem1/2(maxX), Enabled Subsystem/5(maxXleft)
  Enabled Subsystem/13(left) -> minXReadSwitch1/2(addr_in1), minXReadSwitch/2(addr_in1)
  minX/1 -> Enabled Subsystem1/1(minX), Enabled Subsystem/3(minXleft)
  Data Type Conversion2/1 -> Enabled Subsystem/8(y)
  Constant2/1 -> minXWriteSwitch/4(we_in)
  Constant1/1 -> maxXWriteSwitch/4(we_in)
  Constant3/1 -> minYWriteSwitch/4(we_in)
  Constant4/1 -> maxYWriteSwitch/4(we_in)
  HV Counter/3 -> Bus Selector/1, ctrl_out/1
  Bus Selector/2 -> Scope/2  "<hStart>"
  Bus Selector/3 -> Scope/3  "<hEnd>"
  Bus Selector/4 -> Scope/4  "<vStart>"
  Bus Selector/5 -> Subsystem1/1(enable), Delay4/1, minXReadSwitch3/3(frame_end), minXSwitch4/5(frame_end), Scope/5, minXReadSwitch/3(frame_end), Subsystem3/1(reset), Subsystem2/1(reset), minXReadSwitch1/3(frame_end)  "<vEnd>"
  minXReadSwitch1/1(addr_out) -> maxXleft/4
  Enabled Subsystem/12(merger_rd_addr) -> minXReadSwitch3/2(addr_in1)
  pixel_in/1 -> pixel_out/1, Enabled Subsystem/2(pixel)
  Subsystem1/1(counter) -> Delay1/1
  Delay1/1 -> Enabled Subsystem/9(frameNum)
  Logical Operator/1 -> Enabled Subsystem1/Enable
  minXReadSwitch/1(addr_out) -> Delay3/1, minX/4
  Delay2/1 -> Logical Operator/1
  Subsystem2/1(counter) -> minY/4
  Subsystem3/1(counter) -> maxY/4
  minY/1 -> Enabled Subsystem1/3(minY)
  maxY/1 -> Enabled Subsystem1/4(maxY)
  minXReadSwitch3/1(addr_out) -> merger/4
  Delay3/1 -> Enabled Subsystem1/6(index)
  Delay4/1 -> Enabled Subsystem/10(frame_end)
  theta/1 -> Enabled Subsystem/6(theta)

== system hwTarget/hwTarget/Segmentation/Northwest Segmentation ==
  NW : Inport
  ctrl_in : Inport  Port=2
  x0 : Outport
  y0 : Outport  Port=2
  x1 : Outport  Port=3
  y1 : Outport  Port=4
  theta : Outport  Port=5
  ctrl_out : Outport  Port=6

== system hwTarget/hwTarget/Segmentation/Southwest Segmentation ==
  SW : Inport
  ctrl_in : Inport  Port=2
  x0 : Outport
  y0 : Outport  Port=2
  x1 : Outport  Port=3
  y1 : Outport  Port=4
  theta : Outport  Port=5
  ctrl_out : Outport  Port=6

== system hwTarget/hwTarget/Segmentation/West Segmentation ==
  W : Inport
  ctrl_in : Inport  Port=2
  x0 : Outport
  y0 : Outport  Port=2
  x1 : Outport  Port=3
  y1 : Outport  Port=4
  theta : Outport  Port=5
  ctrl_out : Outport  Port=6

== system hwTarget/hwTarget/CordicAtan/CORDIC Algorithm/Iteration_1 ==
  xo : Inport
  yo : Inport  Port=2
  zo : Inport  Port=3
  Add : Sum
  Add1 : Sum  OutDataTypeStr=fixdt(1,NUM_OF_BITS, NUM_OF_BITS-3)
  Add2 : Sum
  cordicLut_3 : Constant  Value=0.463647609000806  OutDataTypeStr=CORDIC_LUT_DT_3  SampleTime=-1
  n_zsign : Subsystem
  n_zsign1 : Subsystem
  zsign : Subsystem
  x : Outport
  y : Outport  Port=2
  z : Outport  Port=3
  wires:
  Add/1 -> z/1
  cordicLut_3/1 -> n_zsign1/2(base)
  zo/1 -> Add/2
  n_zsign1/1(out) -> Add/1
  yo/1 -> zsign/2(base), zsign/1(signof), n_zsign/1(signof), Add2/2
  zsign/1(out) -> Add1/2  "xo"
  xo/1 -> n_zsign/2(base), Add1/1
  Add1/1 -> x/1
  n_zsign/1(out) -> Add2/1
  Add2/1 -> n_zsign1/1(signof), y/1

== system hwTarget/hwTarget/CordicAtan/CORDIC Algorithm/Iteration_10 ==
  xo : Inport
  yo : Inport  Port=2
  zo : Inport  Port=3
  Add : Sum
  X_Logic : Subsystem
  Y_Logic : Subsystem
  cordicLut_12 : Constant  Value=0.000976562189559320  OutDataTypeStr=CORDIC_LUT_DT_12  SampleTime=-1
  n_zsign : Subsystem
  x : Outport
  y : Outport  Port=2
  z : Outport  Port=3
  wires:
  Add/1 -> z/1
  cordicLut_12/1 -> n_zsign/2(base)
  zo/1 -> Add/2
  n_zsign/1(out) -> Add/1
  yo/1 -> Y_Logic/2(yo), X_Logic/2(yo)
  xo/1 -> Y_Logic/1(xo), X_Logic/1(xo)
  X_Logic/1(x) -> x/1
  Y_Logic/1(y) -> n_zsign/1(signof), y/1

== system hwTarget/hwTarget/CordicAtan/CORDIC Algorithm/Iteration_2 ==
  xo : Inport
  yo : Inport  Port=2
  zo : Inport  Port=3
  Add : Sum
  X_Logic : Subsystem
  Y_Logic : Subsystem
  cordicLut_4 : Constant  Value=0.244978663126864  OutDataTypeStr=CORDIC_LUT_DT_4  SampleTime=-1
  n_zsign : Subsystem
  x : Outport
  y : Outport  Port=2
  z : Outport  Port=3
  wires:
  Add/1 -> z/1
  cordicLut_4/1 -> n_zsign/2(base)
  zo/1 -> Add/2
  n_zsign/1(out) -> Add/1
  yo/1 -> Y_Logic/2(yo), X_Logic/2(yo)
  xo/1 -> Y_Logic/1(xo), X_Logic/1(xo)
  X_Logic/1(x) -> x/1
  Y_Logic/1(y) -> n_zsign/1(signof), y/1

== system hwTarget/hwTarget/CordicAtan/CORDIC Algorithm/Iteration_3 ==
  xo : Inport
  yo : Inport  Port=2
  zo : Inport  Port=3
  Add : Sum
  X_Logic : Subsystem
  Y_Logic : Subsystem
  cordicLut_5 : Constant  Value=0.124354994546761  OutDataTypeStr=CORDIC_LUT_DT_5  SampleTime=-1
  n_zsign : Subsystem
  x : Outport
  y : Outport  Port=2
  z : Outport  Port=3
  wires:
  Add/1 -> z/1
  cordicLut_5/1 -> n_zsign/2(base)
  zo/1 -> Add/2
  n_zsign/1(out) -> Add/1
  yo/1 -> Y_Logic/2(yo), X_Logic/2(yo)
  xo/1 -> Y_Logic/1(xo), X_Logic/1(xo)
  X_Logic/1(x) -> x/1
  Y_Logic/1(y) -> n_zsign/1(signof), y/1

== system hwTarget/hwTarget/CordicAtan/CORDIC Algorithm/Iteration_4 ==
  xo : Inport
  yo : Inport  Port=2
  zo : Inport  Port=3
  Add : Sum
  X_Logic : Subsystem
  Y_Logic : Subsystem
  cordicLut_6 : Constant  Value=0.0624188099959574  OutDataTypeStr=CORDIC_LUT_DT_6  SampleTime=-1
  n_zsign : Subsystem
  x : Outport
  y : Outport  Port=2
  z : Outport  Port=3
  wires:
  Add/1 -> z/1
  cordicLut_6/1 -> n_zsign/2(base)
  zo/1 -> Add/2
  n_zsign/1(out) -> Add/1
  yo/1 -> Y_Logic/2(yo), X_Logic/2(yo)
  xo/1 -> Y_Logic/1(xo), X_Logic/1(xo)
  X_Logic/1(x) -> x/1
  Y_Logic/1(y) -> n_zsign/1(signof), y/1

== system hwTarget/hwTarget/CordicAtan/CORDIC Algorithm/Iteration_5 ==
  xo : Inport
  yo : Inport  Port=2
  zo : Inport  Port=3
  Add : Sum
  X_Logic : Subsystem
  Y_Logic : Subsystem
  cordicLut_7 : Constant  Value=0.0312398334302683  OutDataTypeStr=CORDIC_LUT_DT_7  SampleTime=-1
  n_zsign : Subsystem
  x : Outport
  y : Outport  Port=2
  z : Outport  Port=3
  wires:
  Add/1 -> z/1
  cordicLut_7/1 -> n_zsign/2(base)
  zo/1 -> Add/2
  n_zsign/1(out) -> Add/1
  yo/1 -> Y_Logic/2(yo), X_Logic/2(yo)
  xo/1 -> Y_Logic/1(xo), X_Logic/1(xo)
  X_Logic/1(x) -> x/1
  Y_Logic/1(y) -> n_zsign/1(signof), y/1

== system hwTarget/hwTarget/CordicAtan/CORDIC Algorithm/Iteration_6 ==
  xo : Inport
  yo : Inport  Port=2
  zo : Inport  Port=3
  Add : Sum
  X_Logic : Subsystem
  Y_Logic : Subsystem
  cordicLut_8 : Constant  Value=0.0156237286204768  OutDataTypeStr=CORDIC_LUT_DT_8  SampleTime=-1
  n_zsign : Subsystem
  x : Outport
  y : Outport  Port=2
  z : Outport  Port=3
  wires:
  Add/1 -> z/1
  cordicLut_8/1 -> n_zsign/2(base)
  zo/1 -> Add/2
  n_zsign/1(out) -> Add/1
  yo/1 -> Y_Logic/2(yo), X_Logic/2(yo)
  xo/1 -> Y_Logic/1(xo), X_Logic/1(xo)
  X_Logic/1(x) -> x/1
  Y_Logic/1(y) -> n_zsign/1(signof), y/1

== system hwTarget/hwTarget/CordicAtan/CORDIC Algorithm/Iteration_7 ==
  xo : Inport
  yo : Inport  Port=2
  zo : Inport  Port=3
  Add : Sum
  X_Logic : Subsystem
  Y_Logic : Subsystem
  cordicLut_9 : Constant  Value=0.00781234106010111  OutDataTypeStr=CORDIC_LUT_DT_9  SampleTime=-1
  n_zsign : Subsystem
  x : Outport
  y : Outport  Port=2
  z : Outport  Port=3
  wires:
  Add/1 -> z/1
  cordicLut_9/1 -> n_zsign/2(base)
  zo/1 -> Add/2
  n_zsign/1(out) -> Add/1
  yo/1 -> Y_Logic/2(yo), X_Logic/2(yo)
  xo/1 -> Y_Logic/1(xo), X_Logic/1(xo)
  X_Logic/1(x) -> x/1
  Y_Logic/1(y) -> n_zsign/1(signof), y/1

== system hwTarget/hwTarget/CordicAtan/CORDIC Algorithm/Iteration_8 ==
  xo : Inport
  yo : Inport  Port=2
  zo : Inport  Port=3
  Add : Sum
  X_Logic : Subsystem
  Y_Logic : Subsystem
  cordicLut_10 : Constant  Value=0.00390623013196697  OutDataTypeStr=CORDIC_LUT_DT_10  SampleTime=-1
  n_zsign : Subsystem
  x : Outport
  y : Outport  Port=2
  z : Outport  Port=3
  wires:
  Add/1 -> z/1
  cordicLut_10/1 -> n_zsign/2(base)
  zo/1 -> Add/2
  n_zsign/1(out) -> Add/1
  yo/1 -> Y_Logic/2(yo), X_Logic/2(yo)
  xo/1 -> Y_Logic/1(xo), X_Logic/1(xo)
  X_Logic/1(x) -> x/1
  Y_Logic/1(y) -> n_zsign/1(signof), y/1

== system hwTarget/hwTarget/CordicAtan/CORDIC Algorithm/Iteration_9 ==
  xo : Inport
  yo : Inport  Port=2
  zo : Inport  Port=3
  Add : Sum
  X_Logic : Subsystem
  Y_Logic : Subsystem
  cordicLut_11 : Constant  Value=0.00195312251647882  OutDataTypeStr=CORDIC_LUT_DT_11  SampleTime=-1
  n_zsign : Subsystem
  x : Outport
  y : Outport  Port=2
  z : Outport  Port=3
  wires:
  Add/1 -> z/1
  cordicLut_11/1 -> n_zsign/2(base)
  zo/1 -> Add/2
  n_zsign/1(out) -> Add/1
  yo/1 -> Y_Logic/2(yo), X_Logic/2(yo)
  xo/1 -> Y_Logic/1(xo), X_Logic/1(xo)
  X_Logic/1(x) -> x/1
  Y_Logic/1(y) -> n_zsign/1(signof), y/1

== system hwTarget/hwTarget/CordicAtan/CORDIC Algorithm/Setup_Stage ==
  iY : Inport
  iX : Inport  Port=2
  Add : Sum  OutDataTypeStr=fixdt(1,NUM_OF_BITS,NUM_OF_BITS-3)
  cordicLut_1 : Constant  Value=1.57079632679490  OutDataTypeStr=CORDIC_LUT_DT_1  SampleTime=-1
  cordicLut_2 : Constant  Value=0.785398163397448  OutDataTypeStr=CORDIC_LUT_DT_2  SampleTime=-1
  n_zsign : Subsystem
  n_zsign1 : Subsystem
  n_zsign2 : Subsystem
  zsign : Subsystem
  xo : Outport
  yo : Outport  Port=2
  zo : Outport  Port=3
  wires:
  cordicLut_1/1 -> n_zsign1/2(base)
  iY/1 -> zsign/2(base), n_zsign1/1(signof), n_zsign/1(signof), zsign/1(signof)
  n_zsign/1(out) -> n_zsign2/1(signof), yo/1  "yo"
  n_zsign1/1(out) -> Add/1  "zo"
  cordicLut_2/1 -> n_zsign2/2(base)
  iX/1 -> n_zsign/2(base)
  n_zsign2/1(out) -> Add/2
  Add/1 -> zo/1  "zo"
  zsign/1(out) -> xo/1  "xo"

== system hwTarget/hwTarget/CordicAtan/CORDIC Algorithm/Special Cases ==
  iX : Inport
  iY : Inport  Port=2
  Compare To Zero : simulink/Logic and Bit Operations/Compare To Zero  relop===  OutDataTypeStr=boolean
  Compare To Zero1 : simulink/Logic and Bit Operations/Compare To Zero  relop===  OutDataTypeStr=boolean
  Logical Operator : Logic  AllPortsSameDT=off  OutDataTypeStr=boolean
  all_zeros : Outport
  wires:
  Compare To Zero1/1 -> Logical Operator/2
  Logical Operator/1 -> all_zeros/1
  iY/1 -> Compare To Zero1/1
  Compare To Zero/1 -> Logical Operator/1
  iX/1 -> Compare To Zero/1

== system hwTarget/hwTarget/GaussianFilter/Symmetric Filter/Row Filter1 ==
  data_in : Inport
  coefficients : Inport  Port=2
  Delay1 : Delay
  Delay2 : Delay
  Demux : Demux  Outputs=[2, 1]
  Product : Product  OutDataTypeStr=cap_1
  Sum : Sum  Inputs=1  AccumDataTypeStr=cap_1  OutDataTypeStr=cap_1
  Symmetry : Subsystem
  Terminator : Terminator
  data_out : Outport
  wires:
  Product/1 -> Delay1/1
  Symmetry/1(data_out) -> Product/2
  Delay1/1 -> Sum/1
  Delay2/1 -> data_out/1
  Sum/1 -> Delay2/1
  data_in/1 -> Symmetry/1(data_in)
  coefficients/1 -> Demux/1
  Demux/1 -> Product/1
  Demux/2 -> Terminator/1

== system hwTarget/hwTarget/GaussianFilter/Symmetric Filter/Row Filter2 ==
  data_in : Inport
  coefficients : Inport  Port=2
  Delay1 : Delay
  Delay2 : Delay
  Demux : Demux  Outputs=[2, 1]
  Product : Product  OutDataTypeStr=cap_1
  Sum : Sum  Inputs=1  AccumDataTypeStr=cap_1  OutDataTypeStr=cap_1
  Symmetry : Subsystem
  Terminator : Terminator
  data_out : Outport
  wires:
  Product/1 -> Delay1/1
  Symmetry/1(data_out) -> Product/2
  Delay1/1 -> Sum/1
  Delay2/1 -> data_out/1
  Sum/1 -> Delay2/1
  data_in/1 -> Symmetry/1(data_in)
  coefficients/1 -> Demux/1
  Demux/1 -> Product/1
  Demux/2 -> Terminator/1

== system hwTarget/hwTarget/GaussianFilter/Symmetric Filter/Row Filter3 ==
  data_in : Inport
  coefficients : Inport  Port=2
  Delay1 : Delay
  Delay2 : Delay
  Demux : Demux  Outputs=[2, 1]
  Product : Product  OutDataTypeStr=cap_1
  Sum : Sum  Inputs=1  AccumDataTypeStr=cap_1  OutDataTypeStr=cap_1
  Symmetry : Subsystem
  Terminator : Terminator
  data_out : Outport
  wires:
  Product/1 -> Delay1/1
  Symmetry/1(data_out) -> Product/2
  Delay1/1 -> Sum/1
  Delay2/1 -> data_out/1
  Sum/1 -> Delay2/1
  data_in/1 -> Symmetry/1(data_in)
  coefficients/1 -> Demux/1
  Demux/1 -> Product/1
  Demux/2 -> Terminator/1

== system hwTarget/hwTarget/GaussianFilter/Symmetric Filter/Verticle Filter ==
  data_in : Inport
  coefficients : Inport  Port=2
  Delay1 : Delay
  Delay2 : Delay
  Demux : Demux  Outputs=[2, 1]
  Product : Product  OutDataTypeStr=cap_1
  Sum : Sum  Inputs=1  AccumDataTypeStr=cap_1  OutDataTypeStr=cap_1
  Symmetry : Subsystem
  Terminator : Terminator
  data_out : Outport
  wires:
  Product/1 -> Delay1/1
  Symmetry/1(data_out) -> Product/2
  Delay1/1 -> Sum/1
  Delay2/1 -> data_out/1
  Sum/1 -> Delay2/1
  data_in/1 -> Symmetry/1(data_in)
  coefficients/1 -> Demux/1
  Demux/1 -> Product/1
  Demux/2 -> Terminator/1

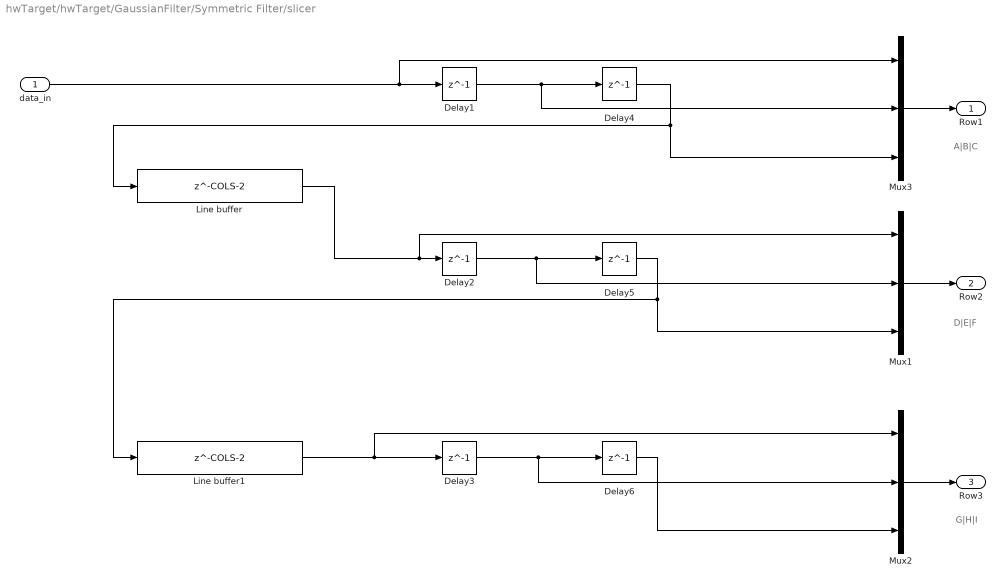
== system hwTarget/hwTarget/GaussianFilter/Symmetric Filter/slicer ==
  note: A|B|C
  note: D|E|F
  note: G|H|I
  data_in : Inport
  Delay{1..6} (6 alike) : Delay  DelayLength=1  InitialCondition=0
  Line buffer : Delay  DelayLength=COLS-2  InitialCondition=0
  Line buffer1 : Delay  DelayLength=COLS-2  InitialCondition=0
  Mux1 : Mux  Inputs=3
  Mux2 : Mux  Inputs=3
  Mux3 : Mux  Inputs=3
  Row1 : Outport  VectorParamsAs1DForOutWhenUnconnected=off
  Row2 : Outport  Port=2  VectorParamsAs1DForOutWhenUnconnected=off
  Row3 : Outport  Port=3  VectorParamsAs1DForOutWhenUnconnected=off
  wires:
  Delay4/1 -> Mux3/3, Line buffer/1
  data_in/1 -> Mux3/1, Delay1/1
  Delay1/1 -> Mux3/2, Delay4/1
  Delay3/1 -> Mux2/2, Delay6/1
  Delay5/1 -> Mux1/3, Line buffer1/1
  Delay6/1 -> Mux2/3
  Line buffer/1 -> Mux1/1, Delay2/1
  Line buffer1/1 -> Mux2/1, Delay3/1
  Delay2/1 -> Mux1/2, Delay5/1
  Mux1/1 -> Row2/1
  Mux2/1 -> Row3/1
  Mux3/1 -> Row1/1

== system hwTarget/hwTarget/Ix//Iy Filters/Ix Filter/Filter ==
  data_in : Inport
  Enable : EnablePort
  Delay : Delay
  Demux : Demux  Outputs=3
  Sum3 : Sum  Inputs=|+-  AccumDataTypeStr=fixdt(1,32,30)  OutDataTypeStr=fixdt(1,32,30)
  Terminator : Terminator
  Terminator1 : Terminator
  Terminator2 : Terminator
  slicer : Subsystem
  data_out : Outport  InitialOutput=0
  wires:
  data_in/1 -> slicer/1(data_in)
  slicer/1(Row1) -> Terminator/1
  slicer/3(Row3) -> Terminator1/1
  slicer/2(Row2) -> Demux/1
  Demux/1 -> Sum3/1
  Demux/3 -> Sum3/2
  Demux/2 -> Terminator2/1
  Delay/1 -> data_out/1
  Sum3/1 -> Delay/1

== system hwTarget/hwTarget/Ix//Iy Filters/Iy Filter/Filter ==
  data_in : Inport
  Enable : EnablePort
  Delay2 : Delay
  Demux : Demux  Outputs=3
  Demux1 : Demux  Outputs=3
  Sum : Sum  Inputs=|+-  AccumDataTypeStr=fixdt(1,32,30)  OutDataTypeStr=fixdt(1,32,30)
  Terminator{,1..4} (5 alike) : Terminator
  slicer : Subsystem
  data_out : Outport  InitialOutput=0
  wires:
  slicer/1(Row1) -> Demux/1
  data_in/1 -> slicer/1(data_in)
  slicer/2(Row2) -> Terminator/1
  slicer/3(Row3) -> Demux1/1
  Demux/1 -> Terminator1/1
  Demux/3 -> Terminator2/1
  Demux/2 -> Sum/1
  Demux1/1 -> Terminator3/1
  Demux1/2 -> Sum/2
  Demux1/3 -> Terminator4/1
  Sum/1 -> Delay2/1
  Delay2/1 -> data_out/1

== system hwTarget/hwTarget/Kirsch Operation North/Binarize/Subsystem ==
  pixel : Inport
  mean : Inport  Port=2
  stddev : Inport  Port=3
  magThrL : Inport  Port=4
  magThrS : Inport  Port=5
  Enable : EnablePort
  Comparator : RelationalOperator  Operator=>  OutDataTypeStr=boolean  RndMeth=Simplest
  Comparator1 : RelationalOperator  Operator=>  OutDataTypeStr=boolean  RndMeth=Simplest
  Delay : Delay  DelayLength=1
  Delay1 : Delay  DelayLength=1
  Delay2 : Delay  DelayLength=1
  MagThrL : Subsystem
  MagThrS : Subsystem
  Out1 : Outport
  Out2 : Outport  Port=2
  wires:
  pixel/1 -> Delay2/1
  MagThrL/1(thresh) -> Delay1/1
  magThrS/1 -> MagThrS/3(dev_step)
  MagThrS/1(thresh) -> Delay/1
  magThrL/1 -> MagThrL/3(dev_step)
  mean/1 -> MagThrS/1(mean), MagThrL/1(mean)
  stddev/1 -> MagThrS/2(stddev), MagThrL/2(stddev)
  Comparator1/1 -> Out2/1
  Comparator/1 -> Out1/1
  Delay/1 -> Comparator1/2
  Delay1/1 -> Comparator/2
  Delay2/1 -> Comparator1/1, Comparator/1
